simulink library "MIL_Test"  (Simulink 6.6)
undefined symbols (not defined in the file or in its folder): getdatatypespecs, slcm, StepSize
libraries: simulink x71, MIL_Test x6
(part 8 of 8)

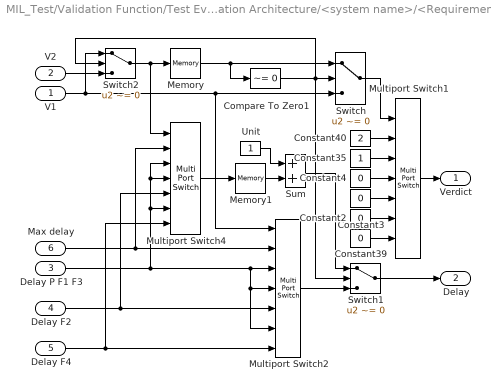
== system MIL_Test/Validation Function/Test Evaluation Architecture/<system name>/<Requirement name>/<Assertions name>/PAS/none - pass - fail/Arbitration/Verdict selection ==
  V1 : Inport
  V2 : Inport  Port=2
  Delay P F1 F3 : Inport  Port=3
  Delay F2 : Inport  Port=4
  Delay F4 : Inport  Port=5
  Max delay : Inport  Port=6
  Compare To Zero1 : simulink/Logic and Bit Operations/Compare To Zero  SystemSampleTime=-1  relop=~=  LogicOutDataTypeMode=boolean  ZeroCross=off
  Constant{2..4,39} (4 alike) : Constant  Value=0
  Constant35 : Constant
  Constant40 : Constant  Value=2
  Memory : Memory
  Memory1 : Memory
  Multiport Switch1 : MultiPortSwitch  Inputs=6  zeroidx=on
  Multiport Switch2 : MultiPortSwitch  Inputs=6  zeroidx=on
  Multiport Switch4 : MultiPortSwitch  Inputs=6  zeroidx=on
  Sum : Sum
  Switch : Switch  Criteria=u2 ~= 0
  Switch1 : Switch  Criteria=u2 ~= 0
  Switch2 : Switch  Criteria=u2 ~= 0
  Unit : Constant
  Verdict : Outport
  Delay : Outport  Port=2
  wires:
  Switch2/1 -> Multiport Switch4/1, Memory/1
  Unit/1 -> Sum/1
  Memory1/1 -> Sum/2
  Sum/1 -> Switch1/1
  Multiport Switch4/1 -> Memory1/1
  Multiport Switch2/1 -> Switch1/3
  Switch1/1 -> Delay/1
  Switch/1 -> Multiport Switch1/1
  Compare To Zero1/1 -> Switch2/2, Switch1/2, Switch/2
  Memory/1 -> Switch/1, Compare To Zero1/1
  Delay F4/1 -> Multiport Switch4/7, Multiport Switch2/7
  Delay F2/1 -> Multiport Switch4/5, Multiport Switch2/5
  Delay P F1 F3/1 -> Multiport Switch4/3, Multiport Switch4/4, Multiport Switch4/6, Multiport Switch2/4, Multiport Switch2/6, Multiport Switch2/3
  Max delay/1 -> Multiport Switch4/2, Multiport Switch2/2
  V1/1 -> Switch2/1, Switch/3, Multiport Switch2/1
  V2/1 -> Switch2/3
  Constant40/1 -> Multiport Switch1/2
  Constant35/1 -> Multiport Switch1/3
  Constant4/1 -> Multiport Switch1/4
  Constant3/1 -> Multiport Switch1/5
  Constant2/1 -> Multiport Switch1/6
  Constant39/1 -> Multiport Switch1/7
  Multiport Switch1/1 -> Verdict/1

== system MIL_Test/Validation Function/Test Evaluation Architecture/<system name>/<Requirement name>/<Assertions name>/PAS/none - pass - fail/Compute delay/Hold1 ==
  " " : Inport
  "    " : Inport  Port=2
  Memory : Memory  Orientation=left
  Switch : Switch  Criteria=u2 ~= 0
  "  " : Outport
  wires:
  " "/1 -> Switch/2
  "    "/1 -> Switch/1
  Switch/1 -> "  "/1, Memory/1
  Memory/1 -> Switch/3

== system MIL_Test/Validation Function/Test Evaluation Architecture/<system name>/<Requirement name>/<Assertions name>/PAS/none - pass - fail/Compute delay1/Hold1 ==
  " " : Inport
  "    " : Inport  Port=2
  Memory : Memory  Orientation=left
  Switch : Switch  Criteria=u2 ~= 0
  "  " : Outport
  wires:
  " "/1 -> Switch/2
  "    "/1 -> Switch/1
  Switch/1 -> "  "/1, Memory/1
  Memory/1 -> Switch/3

== system MIL_Test/Validation Function/Test Evaluation Architecture/<system name>/<Requirement name>/<Assertions name>/PAS/none - pass - fail/Compute delay2/Hold1 ==
  " " : Inport
  "    " : Inport  Port=2
  Memory : Memory  Orientation=left
  Switch : Switch  Criteria=u2 ~= 0
  "  " : Outport
  wires:
  Memory/1 -> Switch/3
  Switch/1 -> Memory/1, "  "/1
  "    "/1 -> Switch/1
  " "/1 -> Switch/2

== stateflow chart Test Control/Test Control Architecture/independent Test Control  ==
  state TestCase1
    entry: TestCase = 1;
  state TestCase2
    entry: TestCase = 2;
  state stop
  (default) -> TestCase1
  TestCase1 -> TestCase2 : after(70, tick)
  TestCase2 -> stop : after(70, tick)
  data: TestCase output double

== stateflow chart Validation Function/Test Evaluation Architecture/Alternative/Alternative Arbitration ==
  state LV1_pass
    en: OverallVerdict=1;
  state LV3_fail
    en: OverallVerdict=0;
  state LV2_inconc
    en: OverallVerdict=2;
  state OV_error
    en: OverallVerdict=10;
  (default) -> (junction 16)
  (junction 16) -> LV1_pass [order 1] : [LocalVerdict1 == 1]
  (junction 16) -> LV2_inconc [order 2] : [LocalVerdict2 == 2 &...
      | LocalVerdict1 ~= 1]
  (junction 16) -> LV3_fail [order 3] : [LocalVerdict3 == 0 & ...
      | LocalVerdict2 ~= 2 &...
      | LocalVerdict1 ~= 1]
  (junction 16) -> OV_error [order 4]
  data: LocalVerdict1 input inherited; LocalVerdict2 input inherited; LocalVerdict3 input inherited; OverallVerdict output double

== matlab function Test Control/Test Control Architecture/Test Control Conditions/IF signal@time1/if false, then TC4 for 200/Embedded MATLAB Function ==
function fcn()
% if u == 1
%signalbuilder('LCTC/Test Stimuli', 'activegroup', 4);
%set_param('LCTC', 'StopTime', '200');
% end

== stateflow chart Validation Function/TODO/User-defined target:  Active_30 ==
  settings: sampleTime=1
  state Inactive/
  state Active/
    entry: aCount = 0
    during: aCount++
    state S1
    state S2
    state S3
    state S4
    (default) -> S1
    S1 -> S2 : [aCount > 10]/t10=1
    S2 -> S3 : [aCount > 20]/t20=1
    S3 -> S4 : [aCount > 30]/t30=1
  Inactive -> Active : [active == 1]
  Active -> Inactive : [active == 0]
  (default) -> Inactive
  data: active input double; aCount local uint32; t10 output double; t20 output double; t30 output double

== stateflow chart Validation Function/TODO/Assertion:  SpeedMaintenance ==
  state Inactive
  state Active
    state OkDiff
    state BigDiff/
      entry: cnt = 0
      during: cnt++
    state Error
    OkDiff -> BigDiff : [diff() > 1]
    BigDiff -> OkDiff [order 2] : [diff() <= 1]
    BigDiff -> Error [order 1] : [cnt > 3]/ok=0
    (default) -> OkDiff
  state d = diff() [function]
    (default) -> (junction 60)
    (junction 60) -> (junction 61) [order 1] : [speed > dSpeed]{d = speed - dSpeed}
    (junction 60) -> (junction 62) [order 2] : {d = dSpeed - speed}
  note: This chart writes 0 to its 'ok' output if vehicle speed ever differs from desired speed by more than 1 for more than
      | 3 seconds while the cruise remains active.  The meaning of the states:
      |
      | Inactive:  chart is in this state if cruise is inactive.
      |
      | Active:  chart is in this state if cruise is active.
      |     Active/OkDiff:  chart is active, difference in speeds <= 1
      |     Active/BigDiff:  chart is active, difference in speeds > 1 for <= 3 seconds
      |     Active/Error:  chart is active, difference in speeds > 1 for > 3 seconds
  (default) -> Inactive : /ok = 1
  Inactive -> Active : [active]
  Active -> Inactive : [!active]
  data: d function_output double; speed input double; dSpeed input double; active input double; cnt local uint32; ok output double =1

== matlab function Test Control/Test Control Architecture/Test Control Conditions/IF signal@time1/if true, then TC2 for 400/Embedded MATLAB Function ==
function fcn()
% if u == 1
%signalbuilder('LCTC/Test Stimuli', 'activegroup', 2);
%set_param('LCTC', 'StopTime', '400');
% end

== matlab function Test Control/Test Control Architecture/Test Control Conditions/IF Signal@SimStopTime for TC = value1/if false, then TC4 for 200/Embedded MATLAB Function ==
function fcn()
% if u == 1
%signalbuilder('LCTC/Test Stimuli', 'activegroup', 4);
%set_param('LCTC', 'StopTime', '200');
% end

== matlab function Test Control/Test Control Architecture/Test Control Conditions/IF Signal@SimStopTime for TC = value1/if true, then TC2 for 400/Embedded MATLAB Function ==
function fcn()
% if u == 1
%signalbuilder('LCTC/Test Stimuli', 'activegroup', 2);
%set_param('LCTC', 'StopTime', '400');
% end

== matlab function Test Control/Test Control Architecture/Connection Helpers/TestControl for TestCases Sequencing NoMask/IF Signal@SimStopTime for TC = value1/if false, then TC4 for 200/Embedded MATLAB Function ==
function fcn()
% if u == 1
%signalbuilder('LCTC/Test Stimuli', 'activegroup', 4);
%set_param('LCTC', 'StopTime', '200');
% end

== matlab function Test Control/Test Control Architecture/Connection Helpers/TestControl for TestCases Sequencing NoMask/IF Signal@SimStopTime for TC = value1/if true, then TC2 for 400/Embedded MATLAB Function ==
function fcn()
% if u == 1
%signalbuilder('LCTC/Test Stimuli', 'activegroup', 2);
%set_param('LCTC', 'StopTime', '400');
% end

== stateflow chart Test Data/Feature generation/Generate feature variants/TestDataVariants Sequence ==
  state TDVariant2
    entry: TDVariant = 2;
  state TDVariant1
    entry: TDVariant = 1;
  TDVariant2 -> TDVariant1 : after(250, tick)
  TDVariant1 -> TDVariant2 : after(250, tick)
  (default) -> TDVariant1
  data: TDVariant output double

== stateflow chart Test Data/Test Data Architecture/<Test data generator>/<Requirement name>/Sequencing of test data in time due to Preconditions ==
  state Precondition1
    state TDataPre1
      entry: TDPre = 1;
    state Init1
      entry: TDPre = 2;
    state Stabilise1
      entry: TDPre = 2;
    Init1 -> TDataPre1 : after(500, tick)
    TDataPre1 -> Stabilise1 : after(1000, tick)
    (default) -> Init1
  state stop
  stop -> Precondition1 : [Activate==1]
  Stabilise1 -> stop : after(500, tick)
  (default) -> Precondition1 : [Activate==1]
  data: Activate input inherited; TDPre output double
